simulink model "NEW_MAIN"  (R2017b)
settings: Solver=VariableStepAuto  StartTime=0.0  StopTime=10.0  RelTol=1e-3
values from neighbouring files (symbols this model uses):
  A = eye(16,16)    [full_input_list.m]
  B = zeros(16,1)    [full_input_list.m]
  C = blkdiag(eye(3,3),zeros(3,3),eye(10,10))    [full_input_list.m]
  currentMax_B = [0;0.8;0.2]    [full_input_list.m]
  deltaT = 0.00001    (= 1e-05)    [full_input_list.m]
  epsilon_UD_slew = .01    (= 0.01)    [full_input_list.m]
  epsilon_UD_spinUp = .01    (= 0.01)    [full_input_list.m]
  freq = 80    [full_input_list.m]    (also in initSimulink.m)
  H = C    [full_input_list.m]
  I_UD = [0.032808359, 0.000617048, 0.000049185;      0.000617048, 0.032531573, 0.000060042;      0.000049185, 0.000060042, 0.007799591]    [full_input_list.m]
  kd = 0.5    [full_input_list.m]    (also in initACS.m = 0.01)
  kd_UD_detumble = 6e-3    (= 0.006)    [full_input_list.m]
  kp = 1    [full_input_list.m]    (also in initACS.m = 0.01)
  magMomentMax_B = sat2CoilArea.*sat2n.*currentMax_B    [full_input_list.m]
  omega_cmd_N = 1e-1*[1 1 -.6]'    [full_input_list.m]
  omega_spinUp_MAG = 0.05    [full_input_list.m]
  OpModes = [0 0 0]    [full_input_list.m]
  OpTimes = [0 1 2]    [full_input_list.m]
  q4_cmd_init = [q4_cmd_init(2:4); q4_cmd_init(1)]    [full_input_list.m]
  Q_k = zeros(16,16)    [full_input_list.m]
  R = R_k    [full_input_list.m]
  sat2CoilArea = 0.8*[0.02; 0.02; 0.01]    [full_input_list.m]
  sat2n = [0; 100; 100]    [full_input_list.m]
  sat2Resistance = sat2WireLength.*sat2WireResistivity./sat2WireArea    [full_input_list.m]
  SeperationTime = 30000    [full_input_list.m]
  spinAxis_B = [1 0 0]    [full_input_list.m]
  u_k = zeros(16,1)    [full_input_list.m]
  w_k = zeros(16,1)    [full_input_list.m]
  Z_k = zeros(16,1)    [full_input_list.m]
undefined symbols (not defined in the file or in its folder): B_n, B_N, DiscIntNeverNeededParam, G_igrf, gyro_DCM_BS, H_igrf, I_B, IAU, Kschmidt, mag_variance, Orbit_time, R_mean, r_n, r_N, v_n, v_N
libraries: aerolibutil x48, vrlib x37, simulink x22, SimMainLibrary x20, dspmathops x6, sharedtransform x4, dspinverses x2, dspmtrx3 x1, aerolibtransform2 x1, aerolibgravity2 x1, lib_violet_env x1
(part 2 of 3)

== system NEW_MAIN/Flight Computers/Center Cube Controller/Torque Coil Management ==
  note: Why does torque coils suddenly become PWM?
  B_N : Inport
  torque_cmd_N : Inport  Port=2
  q : Inport  Port=3
  Calculate Coil Torque and Current : Subsystem
  Constant4 : Constant  Value=sat2CoilArea.*sat2n.*currentMax_B
  Magnetic Moment Unit Vector : Subsystem
  Magnetic Moment Vector : Subsystem
  Product2 : Product
  Quaternion Rotation : aerolibutil/Quaternion Rotation
  Reduce Wasted Effort : Subsystem
  Saturation : Saturate  Commented=on  UpperLimit=magMomentMax_B(2:3)  LowerLimit=-magMomentMax_B(2:3)
  Selector : Selector  InputPortWidth=3  IndexOptions=Index vector (dialog)  Indices=[2 3]  OutputSizes=1
  Vector Saturation1 : SimMainLibrary/Vector Saturation
      settings: SourceProductName=CUGravity Library
  torque : Constant  Commented=on  Value=[0;1;-1]
  torque_coils : Outport
  CenterCube_PWM_cmds : Outport  Port=2
  wires:
  Constant4/1 -> Selector/1
  B_N/1 -> Calculate Coil Torque and Current/4(B_N), Quaternion Rotation/2
  q/1 -> Quaternion Rotation/1, Calculate Coil Torque and Current/3(q), Magnetic Moment Unit Vector/2(q)
  Reduce Wasted Effort/1(mu_sat_B1) -> Calculate Coil Torque and Current/2(mu_B23)  "mu_B23"
  Vector Saturation1/1 -> Reduce Wasted Effort/2(mu_sat_B)  "mu_sat_B"
  torque_cmd_N/1 -> Magnetic Moment Vector/2(torque_cmd_N), Calculate Coil Torque and Current/1(torque_cmd_N), Magnetic Moment Unit Vector/1(torque_cmd_N)  "torque_cmd_N"
  Magnetic Moment Unit Vector/1(muHat_B) -> Magnetic Moment Vector/1(muHat_B), Reduce Wasted Effort/1(muHat_B)
  Quaternion Rotation/1 -> Reduce Wasted Effort/3(B_B), Magnetic Moment Vector/3(B_B)  "B_B"
  Product2/1 -> torque_coils/1
  Magnetic Moment Vector/1(mu_raw_B) -> Vector Saturation1/1  "mu_raw_B"
  Calculate Coil Torque and Current/1(torque_N) -> Product2/1
  Calculate Coil Torque and Current/2(Sign_B & mu) -> Product2/2
  Calculate Coil Torque and Current/3(coils_I) -> CenterCube_PWM_cmds/1
  Selector/1 -> Vector Saturation1/2

== system NEW_MAIN/Flight Computers/CenterCube EKF/Kalman Gain and Estamated State Computation ==
  P_kp : Inport
  x_kp : Inport  Port=2
  Y : Inport  Port=3
  " LU Inverse" : dspinverses/ LU Inverse
      settings: SourceProductName=DSP System Toolbox
  Add1 : Sum
  Add2 : Sum
  Add3 : Sum  Inputs=-+
  H : Constant  Value=H
  H1 : Constant  Value=H
  Math Function : Math  Operator=transpose  SaturateOnIntegerOverflow=on
  Product{,1,3..4,6} (5 alike) : Product  Multiplication=Matrix(*)
  Product2 : Product
  R : Constant  Value=R
  K : Outport
  x_k : Outport  Port=2
  wires:
  H/1 -> Product3/1, Product1/2, Math Function/1
  " LU Inverse"/1 -> Product/2
  Product1/1 -> Product/1
  Math Function/1 -> Product4/2
  Product/1 -> Product2/1, K/1  "Kalman Gain K"
  x_kp/1 -> Add2/1, Product6/2
  Y/1 -> Add3/2
  R/1 -> Add1/2
  Product4/1 -> Add1/1
  Add1/1 -> " LU Inverse"/1
  Product3/1 -> Product4/1
  H1/1 -> Product6/1
  Product6/1 -> Add3/1
  P_kp/1 -> Product3/2, Product1/1
  Add2/1 -> x_k/1
  Add3/1 -> Product2/2
  Product2/1 -> Add2/2

== system NEW_MAIN/Flight Computers/CenterCube EKF/New State Prediction  ==
  note: LKF
  note: EKF
  P_k-1 : Inport
  x_k-1 : Inport  Port=2
  A_LKF : Subsystem
  Add1 : Sum  Inputs=+++
  Add2 : Sum
  Add3 : Sum
  B : Constant  Value=B
  Math Function : Math  Operator=transpose  SaturateOnIntegerOverflow=on
  Math Function1 : Math  Operator=transpose  SaturateOnIntegerOverflow=on
  Predictions : MATLAB Function  TreatAsAtomicUnit=on
  Product{,1..5} (6 alike) : Product  Multiplication=Matrix(*)
  Q_k : Constant  Value=Q_k
  Q_k1 : Constant  Value=Q_k
  Terminator2 : Terminator
  Terminator3 : Terminator
  u_k : Constant  Value=u_k
  w_k : Constant  Value=w_k
  P_kp : Outport
  "x_kp  " : Outport  Port=2
  wires:
  Product2/1 -> Product3/1
  Math Function/1 -> Product3/2
  Product/1 -> Add1/1
  B/1 -> Product1/1
  Product1/1 -> Add1/2
  u_k/1 -> Product1/2
  w_k/1 -> Add1/3
  Q_k/1 -> Add2/2
  P_k-1/1 -> [A], Product2/2
  Product3/1 -> Add2/1
  x_k-1/1 -> Predictions/1(x_ko), Product/2, A_LKF/1(In1)
  A_LKF/1(Out1) -> Product2/1, Math Function/1, Product/1  "A"
  Predictions/1(F) -> Math Function1/1, Product4/1
  [A] -> Product4/2
  Product4/1 -> Product5/1
  Math Function1/1 -> Product5/2
  Predictions/2(x_kp) -> "x_kp  "/1  "x_kps"
  Product5/1 -> Add3/1
  Q_k1/1 -> Add3/2
  Add3/1 -> P_kp/1  "P_kp"
  Add2/1 -> Terminator2/1  "P_kp"
  Add1/1 -> Terminator3/1  "x_kp"

== system NEW_MAIN/Flight Computers/CenterCube EKF/Y computation ==
  In1 : Inport
  Add2 : Sum
  C : Constant  Value=C
  Product2 : Product  Multiplication=Matrix(*)
  "Z_k " : Constant  Value=Z_k
  Y : Outport
  wires:
  Add2/1 -> Y/1
  "Z_k "/1 -> Add2/2
  In1/1 -> Product2/2
  C/1 -> Product2/1
  Product2/1 -> Add2/1

== system NEW_MAIN/Flight Computers/CenterCube EKF/x_measured ==
  Sensor_data : Inport
  Bus Selector1 : BusSelector  OutputSignals=w_BN_1,magnetometer_1,sun_B,r_LLA,accelerometer_1,time
  Constant : Constant  Value=[0;0;0]
  Lookup Tables : Subsystem
  Terminator : Terminator
  Vector Concatenate : Concatenate  NumInputs=5
  q_N from Sensors : Subsystem
  x_measured : Outport
  B_N : Outport  Port=2
  wires:
  Bus Selector1/4 -> Vector Concatenate/1, Lookup Tables/1(x_pos)  "<r_LLA>"
  Vector Concatenate/1 -> x_measured/1
  Lookup Tables/2(V_sun_N) -> q_N from Sensors/4(V_sun_N)
  Bus Selector1/3 -> q_N from Sensors/2(V_sun_B)  "<sun_B>"
  Lookup Tables/1(B_N) -> B_N/1, q_N from Sensors/3(B_N)
  q_N from Sensors/2(Q) -> Terminator/1
  Sensor_data/1 -> Bus Selector1/1
  Bus Selector1/1 -> Vector Concatenate/4  "<w_BN_1>"
  Constant/1 -> Vector Concatenate/2  "xdot_measured"
  Bus Selector1/5 -> Vector Concatenate/3  "<accelerometer_1>"
  q_N from Sensors/1(q_N) -> Vector Concatenate/5  "quat_measured"
  Bus Selector1/2 -> q_N from Sensors/1(B_B)  "<magnetometer_1>"
  Bus Selector1/6 -> Lookup Tables/2(time)  "<time>"

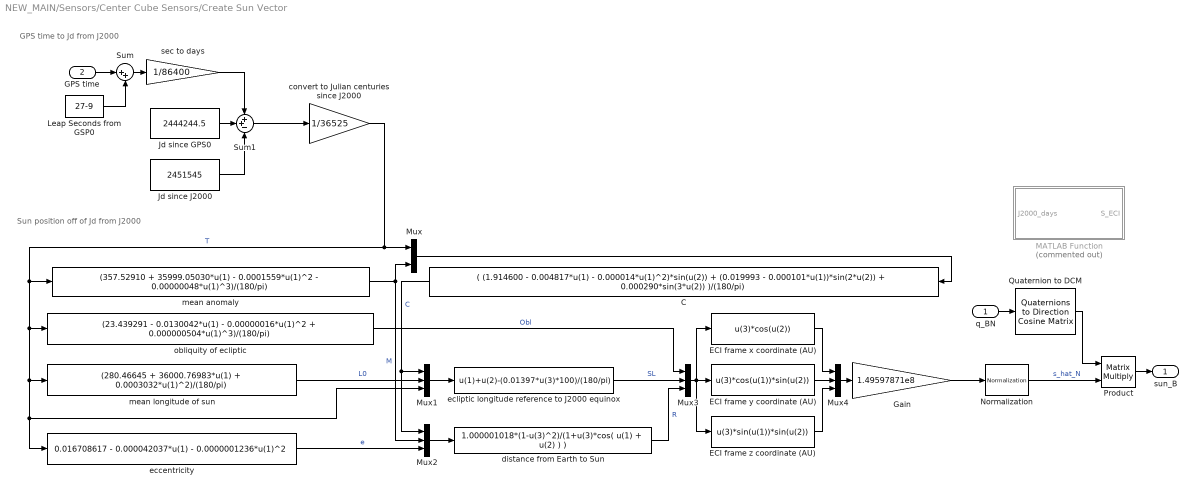
== system NEW_MAIN/Sensors/Center Cube Sensors/Create Sun Vector ==
  note: Sun position off of
      | Jd from J2000
  note: GPS time to
      | Jd from J2000
  q_BN : Inport
  GPS time : Inport  Port=2
  C : Fcn  Expr=( (1.914600 - 0.004817*u(1) - 0.000014*u(1)^2)*sin(u(2)) + (0.019993 - 0.000101*u(1))*sin(2*u(2)) + 0.000290*sin(3*u(2)) )/(180/pi)
  "ECI frame x coordinate (AU) " : Fcn  Expr=u(3)*cos(u(2))
  "ECI frame y coordinate (AU) " : Fcn  Expr=u(3)*cos(u(1))*sin(u(2))
  "ECI frame z coordinate (AU) " : Fcn  Expr=u(3)*sin(u(1))*sin(u(2))
  Gain : Gain  Gain=1.49597871e8
  Jd since GPS0 : Constant  Value=2444244.5
  Jd since J2000 : Constant  Value=2451545
  "Leap Seconds from GSP0 " : Constant  Value=27-9
  MATLAB Function : MATLAB Function  Commented=on  TreatAsAtomicUnit=on
  Mux : Mux  Inputs=2
  Mux{1..4} (4 alike) : Mux  Inputs=3
  Normalization : dspmathops/Normalization  NormType=2-norm  Bias=1e-10  NormOver=Each column  Dimension=1  outputDataTypeStr=Inherit: Same as product output  outputLastDataTypeStr=Inherit: Same as product output  outputMin=[]  outputMax=[]  accumDataTypeStr=Inherit: Same as product output  accumLastDataTypeStr=Inherit: Same as product output  roundingMode=Floor  overflowMode=off
      settings: SourceProductName=DSP System Toolbox
  Product : Product  Multiplication=Matrix(*)
  Quaternion to DCM : sharedtransform/Quaternions to  Direction Cosine Matrix
      settings: SourceProductName=Aerospace Blockset  SourceProductBaseCode=AE
  Sum : Sum  Inputs=|++
  Sum1 : Sum  Inputs=++-
  convert to Julian centuries since J2000 : Gain  Gain=1/36525
  distance from Earth to Sun : Fcn  Expr=1.000001018*(1-u(3)^2)/(1+u(3)*cos( u(1) + u(2) ) )
  eccentricity : Fcn  Expr=0.016708617 - 0.000042037*u(1) - 0.0000001236*u(1)^2
  ecliptic longitude reference to J2000 equinox : Fcn  Expr=u(1)+u(2)-(0.01397*u(3)*100)/(180/pi)
  mean anomaly : Fcn  Expr=(357.52910 + 35999.05030*u(1) - 0.0001559*u(1)^2 - 0.00000048*u(1)^3)/(180/pi)
  mean longitude of sun : Fcn  Expr=(280.46645 + 36000.76983*u(1) + 0.0003032*u(1)^2)/(180/pi)
  obliquity of ecliptic : Fcn  Expr=(23.439291 - 0.0130042*u(1) - 0.00000016*u(1)^2 + 0.000000504*u(1)^3)/(180/pi)
  sec to days : Gain  Gain=1/86400
  sun_B : Outport
  wires:
  Product/1 -> sun_B/1
  q_BN/1 -> Quaternion to DCM/1
  Normalization/1 -> Product/2  "s_hat_N"
  Quaternion to DCM/1 -> Product/1
  Gain/1 -> Normalization/1
  Jd since J2000/1 -> Sum1/3
  Jd since GPS0/1 -> Sum1/2
  sec to days/1 -> Sum1/1
  Sum/1 -> sec to days/1
  "Leap Seconds from GSP0 "/1 -> Sum/2
  GPS time/1 -> Sum/1
  Mux3/1 -> "ECI frame z coordinate (AU) "/1, "ECI frame y coordinate (AU) "/1, "ECI frame x coordinate (AU) "/1
  obliquity of ecliptic/1 -> Mux3/1  "Obl"
  distance from Earth to Sun/1 -> Mux3/3  "R"
  Mux2/1 -> distance from Earth to Sun/1
  ecliptic longitude reference to J2000 equinox/1 -> Mux3/2  "SL"
  eccentricity/1 -> Mux2/3  "e"
  mean anomaly/1 -> Mux2/2, Mux/2  "M"
  C/1 -> Mux2/1, Mux1/1  "C"
  Mux1/1 -> ecliptic longitude reference to J2000 equinox/1
  Mux/1 -> C/1
  mean longitude of sun/1 -> Mux1/2  "L0"
  convert to Julian centuries since J2000/1 -> eccentricity/1, Mux1/3, mean longitude of sun/1, obliquity of ecliptic/1, mean anomaly/1, Mux/1  "T"
  Sum1/1 -> convert to Julian centuries since J2000/1
  "ECI frame y coordinate (AU) "/1 -> Mux4/2
  "ECI frame x coordinate (AU) "/1 -> Mux4/1
  "ECI frame z coordinate (AU) "/1 -> Mux4/3
  Mux4/1 -> Gain/1

== system NEW_MAIN/Sensors/Center Cube Sensors/GPS ==
  note: Position in the sensor reference frame
  note: GPS Sensor Spoofing
      | We must specify the GPS variance and seed later when we have more time
      |
      | DCM of ECFE wrt ECI is not filled in
      |
      | GPS start time needs to be filled in.
      |
      | Violet was able to check for corrupt signals - that is the next step
  note: Velocity in the sensor reference frame
  r_N : Inport
  v_N : Inport  Port=2
  DCM of ECFC wrt ECI : Constant  Value=eye(3)
  DCM of ECFC wrt ECI1 : Constant  Value=eye(3)
  Digital Clock : DigitalClock
  GPS start time : Constant  Value=0
  Position random noise : RandomNumber  SampleTime=0.1
  Product : Product
  Product1 : Product
  Sum : Sum
  Sum1 : Sum
  Sum2 : Sum  Inputs=|++
  Velocity random noise : RandomNumber  SampleTime=0.1
  r_S : Outport
  v_S : Outport  Port=2
  Time : Outport  Port=3
  wires:
  Sum/1 -> r_S/1
  Position random noise/1 -> Sum/2
  Sum1/1 -> v_S/1
  Velocity random noise/1 -> Sum1/2
  GPS start time/1 -> Sum2/1
  Digital Clock/1 -> Sum2/2
  Sum2/1 -> Time/1
  DCM of ECFC wrt ECI/1 -> Product/1
  r_N/1 -> Product/2
  Product/1 -> Sum/1
  DCM of ECFC wrt ECI1/1 -> Product1/1
  v_N/1 -> Product1/2
  Product1/1 -> Sum1/1

== system NEW_MAIN/Sensors/Center Cube Sensors/Gyro ==
  note: Gyro Sensor Spoofing
      |
      | Lots of work left to be done on the Gyro. Violet tracks the gyro bias - necessary?
      |
      | Violet also records the time of the gyro - is this simply a diagnostic step?
  w_BN_B : Inport
  Bias : MATLAB Function  TreatAsAtomicUnit=on
  Bus Creator : BusCreator  Inputs=2
  Digital Clock : DigitalClock
  Discrete-Time Integrator : DiscreteIntegrator  gainval=1  InitialConditionSetting=State (most efficient)  ICPrevOutput=DiscIntNeverNeededParam  ICPrevScaledInput=DiscIntNeverNeededParam
  Gyro_DCM_BS : Constant  Value=gyro_DCM_BS
  Product : Product  Multiplication=Matrix(*)
  Random Bias Steps : RandomNumber  SampleTime=0.1
  Random Noise : RandomNumber  SampleTime=0.1
  Sum : Sum
  w_SN_S_m : Outport
  time : Outport  Port=2
  Gyro : Outport  Port=3
  wires:
  w_BN_B/1 -> Product/2
  Random Bias Steps/1 -> Discrete-Time Integrator/1
  Product/1 -> Sum/1
  Discrete-Time Integrator/1 -> Sum/2
  Sum/1 -> Bias/1(w)
  Random Noise/1 -> Bias/2(noise)
  Bias/1(wn) -> Bus Creator/1, w_SN_S_m/1
  Gyro_DCM_BS/1 -> Product/1
  Digital Clock/1 -> Bus Creator/2, time/1
  Bus Creator/1 -> Gyro/1

== system NEW_MAIN/Sensors/Center Cube Sensors/Magnetometer ==
  note: Teslas to Gauss
  note: from r_E to b_B is in Violet Dynamics Block.
      | The rest is in their sensor block.
  note: b_B
  note: DCM of Body wrt Neutral
  note: Pulled from NASA Langley
  note: The block takes the magnetic field in the body reference frame
      | and transforms it into magnetic field in the sensor reference
      | frame.
      |
      | We still need the DCM and the variance of the magnetometer
  r_E : Inport  PortDimensions=[1 3]
  Bus Creator : BusCreator  Inputs=2
  DCM B wrt S : Constant  Value=eye(3)
  DCM of BN : Constant  Value=eye(3)
  DCM of ECFC wrt ECI : Constant  Value=eye(3)
  Digital Clock : DigitalClock
  Gain : Gain  Gain=1e4
  Magnetic Field Model : Subsystem
  Math Function : Math  Operator=transpose  SaturateOnIntegerOverflow=on
  Math Function1 : Math  Operator=transpose  SaturateOnIntegerOverflow=on
  Matrix Multiply : Product  Multiplication=Matrix(*)
  Matrix Multiply1 : Product  Multiplication=Matrix(*)
  Product : Product  Multiplication=Matrix(*)
  Random Number : RandomNumber  Variance=mag_variance  SampleTime=0.1
  Sine Wave : Sin  Amplitude=0 * 1e-6 * randn(3, 1)  Frequency=2*pi / (90 * 60)  SampleTime=0
  Sum : Sum  Inputs=|++
  Sum1 : Sum  Inputs=|++
  b_S : Outport
  Time : Outport  Port=2
  Magnetometer : Outport  Port=3
  wires:
  Matrix Multiply1/1 -> Sum/1
  Random Number/1 -> Sum/2
  DCM B wrt S/1 -> Math Function/1
  Sum/1 -> Product/2
  Math Function/1 -> Product/1
  Product/1 -> Gain/1
  Gain/1 -> Bus Creator/1, b_S/1
  r_E/1 -> Magnetic Field Model/1(r_E)
  Magnetic Field Model/1(b_E) -> Sum1/1
  Sine Wave/1 -> Sum1/2
  Sum1/1 -> Matrix Multiply/2
  Math Function1/1 -> Matrix Multiply/1
  Matrix Multiply/1 -> Matrix Multiply1/2
  DCM of ECFC wrt ECI/1 -> Math Function1/1
  DCM of BN/1 -> Matrix Multiply1/1
  Digital Clock/1 -> Bus Creator/2, Time/1
  Bus Creator/1 -> Magnetometer/1

== system NEW_MAIN/Sensors/Center Cube Sensors/Sun Sensor ==
  In1 : Inport
  Out1 : Outport
  wires:
  In1/1 -> Out1/1

== system NEW_MAIN/Flight Computers/Center Cube Controller/SafeMode/STATUS_MODE_DETERMINATION/ATTITUDE_COMPENSATOR_OLD.TorqueD ==
  note: Regulator
      | - q_target = <input>
      | - w_target = [0 0 0]
  note: Derivative Controller
      | This controller is a pure derivative controller. It calculates torque to purely oppose the angular velocity. It is better behaved in the short-run than a PD controller projected onto the B field normal plane, but it does not allow for a quaternion command, only a detumble to an unknown attitude.
  note: Markley Regulator
      | This regulator takes the current directional quaterion vector, the target quaterion, the intertial matrix, and the current angular velocity to determine the required torque necessary to the slew.
      |
      | The equation is 7.8 listed on page 290 of Fundamentals of Spacecraft Attitude Determination and Control. The input I is currently not defined. Also important to the equation is equation 7.2
  w_BN_N : Inport
  I_B : Inport  Port=2
  q : Inport  Port=3
  f : TriggerPort  TriggerType=function-call  VariantControl=(inherit)
      settings: CopyFcn=Stateflow.SLINSF.SimulinkMan.removeBlockPreDeleteFcn  PreDeleteFcn=Stateflow.SLINSF.SimulinkMan.unsafePredeleteFcn
  Display : Display
  Display3 : Display
  Gain3 : Gain  Gain=kd_UD_detumble
  Gain5 : Gain  Gain=-1
  Gain6 : Gain  Commented=on  Gain=1/I_B(1,1)
  Math Function : Math  Operator=transpose  SaturateOnIntegerOverflow=on
  Product2 : Product  Multiplication=Matrix(*)
  Product3 : Product  Inputs=3  Multiplication=Matrix(*)
  Q_B_N : Display
  Quaternions to Direction Cosine Matrix : sharedtransform/Quaternions to  Direction Cosine Matrix
      settings: SourceProductName=Aerospace Blockset  SourceProductBaseCode=AE
  Scope : Scope
  T_N : Outport
  wires:
  Math Function/1 -> Product3/1
  q/1 -> Quaternions to Direction Cosine Matrix/1, Scope/1
  Product3/1 -> Product2/1, Display/1  "I_N"
  Quaternions to Direction Cosine Matrix/1 -> Q_B_N/1, Product3/3, Math Function/1
  Gain3/1 -> T_N/1  "torque_N"
  I_B/1 -> Product3/2, Display3/1
  Gain5/1 -> Gain3/1
  w_BN_N/1 -> Product2/2  "w_BN_N"
  Product2/1 -> Gain5/1

== system NEW_MAIN/Flight Computers/Center Cube Controller/SafeMode/STATUS_MODE_DETERMINATION/ATTITUDE_COMPENSATOR_OLD.TorqueDeployed ==
  note: Regulator
      | - q_target = [0 0 0 1]
      | - w_target = [0 0 0]
  q : Inport
  w_BN_N : Inport  Port=2
  f : TriggerPort  TriggerType=function-call  VariantControl=(inherit)
      settings: CopyFcn=Stateflow.SLINSF.SimulinkMan.removeBlockPreDeleteFcn  PreDeleteFcn=Stateflow.SLINSF.SimulinkMan.unsafePredeleteFcn
  Add : Sum
  Gain : Gain  Gain=-1
  Gain1 : Gain  Gain=kp
  Gain2 : Gain  Gain=-1
  Gain3 : Gain  Gain=kd
  Quaternion Inverse : aerolibutil/Quaternion Inverse
      settings: SourceProductName=Aerospace Blockset
  Quaternion Multiplication : aerolibutil/Quaternion Multiplication
  Selector : Selector  InputPortWidth=4  IndexOptions=Index vector (dialog)  Indices=[1 2 3]  OutputSizes=1
  Target q : Constant  Value=[ 0 0 0 1 ]
  T_N : Outport
  wires:
  Gain1/1 -> Gain/1
  Gain2/1 -> Add/2
  Gain/1 -> Add/1
  w_BN_N/1 -> Gain3/1
  Quaternion Inverse/1 -> Quaternion Multiplication/2
  Gain3/1 -> Gain2/1
  Add/1 -> T_N/1
  q/1 -> Quaternion Multiplication/1
  Selector/1 -> Gain1/1
  Quaternion Multiplication/1 -> Selector/1
  Target q/1 -> Quaternion Inverse/1

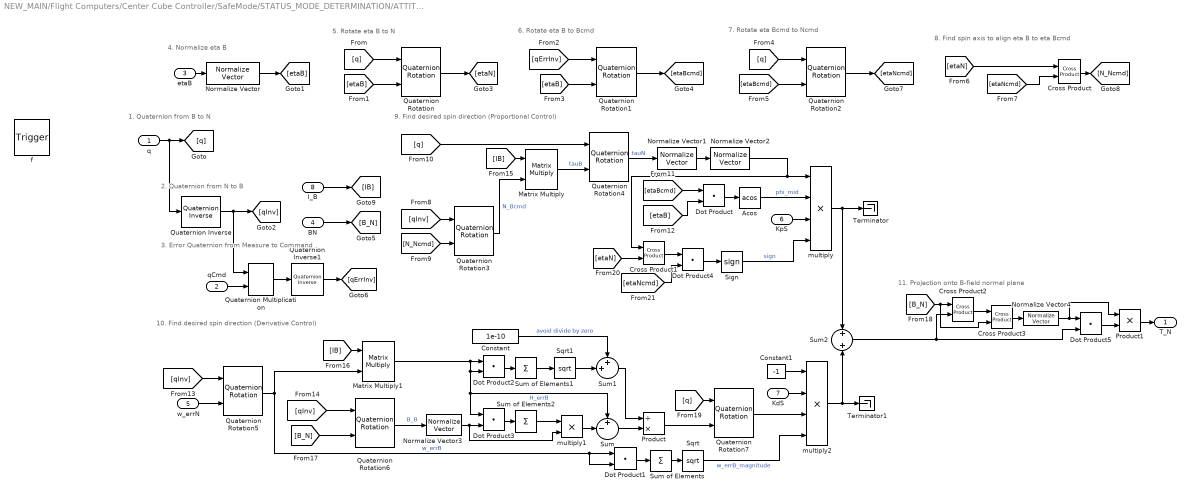
== system NEW_MAIN/Flight Computers/Center Cube Controller/SafeMode/STATUS_MODE_DETERMINATION/ATTITUDE_COMPENSATOR_OLD.TorquePD_Slew ==
  note: 9. Find desired spin direction (Proportional Control)
  note: 10. Find desired spin direction (Derivative Control)
  note: 4. Normalize eta B
  note: 5. Rotate eta B to N
  note: 6. Rotate eta B to Bcmd
  note: 7. Rotate eta Bcmd to Ncmd
  note: 8. Find spin axis to align eta B to eta Bcmd
  note: 1. Quaternion from B to N
  note: 3. Error Quaternion from Measure to Command
  note: 2. Quaternion from N to B
  note: 11. Projection onto B-field normal plane
  q : Inport
  qCmd : Inport  Port=2
  etaB : Inport  Port=3
  BN : Inport  Port=4
  w_errN : Inport  Port=5
  KpS : Inport  Port=6
  KdS : Inport  Port=7
  I_B : Inport  Port=8
  f : TriggerPort  TriggerType=function-call  VariantControl=(inherit)
      settings: CopyFcn=Stateflow.SLINSF.SimulinkMan.removeBlockPreDeleteFcn  PreDeleteFcn=Stateflow.SLINSF.SimulinkMan.unsafePredeleteFcn
  Acos : Trigonometry  Operator=acos
  Constant : Constant  Value=1e-10
  Constant1 : Constant  Value=-1
  Cross Product{,1..3} (4 alike) : vrlib/Utilities/Cross Product
      settings: SourceProductBaseCode=VR
  Dot Product{,1..5} (6 alike) : DotProduct  InputSameDT=on  OutDataTypeStr=Inherit: Inherit via internal rule
  Matrix Multiply : Product  Multiplication=Matrix(*)
  Matrix Multiply1 : Product  Multiplication=Matrix(*)
  Normalize Vector{,1..4} (5 alike) : vrlib/Utilities/Normalize Vector  maxzero=0
      settings: SourceProductName=Simulink 3D Animation  SourceProductBaseCode=VR
  Product : Product  Inputs=/*
  Product1 : Product
  Quaternion Inverse : aerolibutil/Quaternion Inverse
      settings: SourceProductName=Aerospace Blockset
  Quaternion Inverse1 : aerolibutil/Quaternion Inverse
      settings: SourceProductName=Aerospace Blockset
  Quaternion Multiplication : aerolibutil/Quaternion Multiplication
  Quaternion Rotation{,1..7} (8 alike) : aerolibutil/Quaternion Rotation
  Sign : Signum
  Sqrt : Sqrt  SaturateOnIntegerOverflow=on
  Sqrt1 : Sqrt  SaturateOnIntegerOverflow=on
  Sum : Sum  Inputs=+-|
  Sum of Elements : Sum  Inputs=+
  Sum of Elements1 : Sum  Inputs=+
  Sum of Elements2 : Sum  Inputs=+
  Sum1 : Sum  Inputs=++|
  Sum2 : Sum
  Terminator : Terminator
  Terminator1 : Terminator
  multiply : Product  Inputs=****
  multiply1 : Product  Inputs=**
  multiply2 : Product  Inputs=****
  T_N : Outport
  wires:
  Cross Product2/1 -> Cross Product3/1
  etaB/1 -> Normalize Vector/1
  Sqrt/1 -> multiply2/4  "w_errB_magnitude"
  [etaBcmd] -> Dot Product/1
  Sum1/1 -> Product/1
  Normalize Vector4/1 -> Product1/1, Dot Product5/1
  multiply/1 -> Terminator/1, Sum2/1
  Sum/1 -> Product/2
  Quaternion Rotation5/1 -> Dot Product1/1, Dot Product1/2, Matrix Multiply1/2  "w_errB"
  multiply2/1 -> Terminator1/1, Sum2/2
  Sign/1 -> multiply/4  "sign"
  Quaternion Rotation2/1 -> [etaNcmd]
  [etaNcmd] -> Dot Product4/2
  Constant1/1 -> multiply2/1
  Quaternion Rotation6/1 -> Normalize Vector3/1  "B_B"
  Sqrt1/1 -> Sum1/2
  Sum of Elements2/1 -> multiply1/1
  Sum of Elements1/1 -> Sqrt1/1
  Dot Product3/1 -> Sum of Elements2/1
  KdS/1 -> multiply2/2
  Quaternion Rotation7/1 -> multiply2/3
  Dot Product1/1 -> Sum of Elements/1
  multiply1/1 -> Sum/2
  Quaternion Rotation1/1 -> [etaBcmd]
  [q] -> Quaternion Rotation4/1
  [etaN] -> Cross Product1/2
  Constant/1 -> Sum1/1  "avoid divide by zero"
  KpS/1 -> multiply/3
  Matrix Multiply1/1 -> Sum/1, Dot Product3/1, Dot Product2/2, Dot Product2/1  "H_errB"
  Cross Product1/1 -> Dot Product4/1
  Normalize Vector1/1 -> Normalize Vector2/1
  Dot Product4/1 -> Sign/1
  Dot Product2/1 -> Sum of Elements1/1
  Dot Product/1 -> Acos/1
  Normalize Vector3/1 -> Dot Product3/2, multiply1/2
  I_B/1 -> [IB]
  [qInv] -> Quaternion Rotation5/1
  [etaB] -> Dot Product/2
  [q] -> Quaternion Rotation/1
  [IB] -> Matrix Multiply1/1
  Quaternion Rotation3/1 -> Matrix Multiply/2  "N_Bcmd"
  [q] -> Quaternion Rotation2/1
  [etaBcmd] -> Quaternion Rotation2/2
  Quaternion Multiplication/1 -> Quaternion Inverse1/1
  Normalize Vector2/1 -> Cross Product1/1, multiply/1
  [qInv] -> Quaternion Rotation6/1
  qCmd/1 -> Quaternion Multiplication/2
  q/1 -> [q], Quaternion Inverse/1
  [etaB] -> Quaternion Rotation1/2
  [etaB] -> Quaternion Rotation/2
  [N_Ncmd] -> Quaternion Rotation3/2
  Quaternion Rotation4/1 -> Normalize Vector1/1  "tauN"
  Quaternion Inverse/1 -> Quaternion Multiplication/1, [qInv]
  [qErrInv] -> Quaternion Rotation1/1
  Matrix Multiply/1 -> Quaternion Rotation4/2  "tauB"
  Cross Product/1 -> [N_Ncmd]
  [B_N] -> Quaternion Rotation6/2
  w_errN/1 -> Quaternion Rotation5/2
  [qInv] -> Quaternion Rotation3/1
  Normalize Vector/1 -> [etaB]
  Product1/1 -> T_N/1
  Quaternion Rotation/1 -> [etaN]
  Quaternion Inverse1/1 -> [qErrInv]
  BN/1 -> [B_N]
  Product/1 -> Quaternion Rotation7/2
  [etaN] -> Cross Product/1
  Acos/1 -> multiply/2  "phi_mid"
  [etaNcmd] -> Cross Product/2
  Cross Product3/1 -> Normalize Vector4/1
  [B_N] -> Cross Product2/1, Cross Product3/2
  Dot Product5/1 -> Product1/2
  [q] -> Quaternion Rotation7/1
  Sum of Elements/1 -> Sqrt/1
  [IB] -> Matrix Multiply/1
  Sum2/1 -> Cross Product2/2, Dot Product5/2

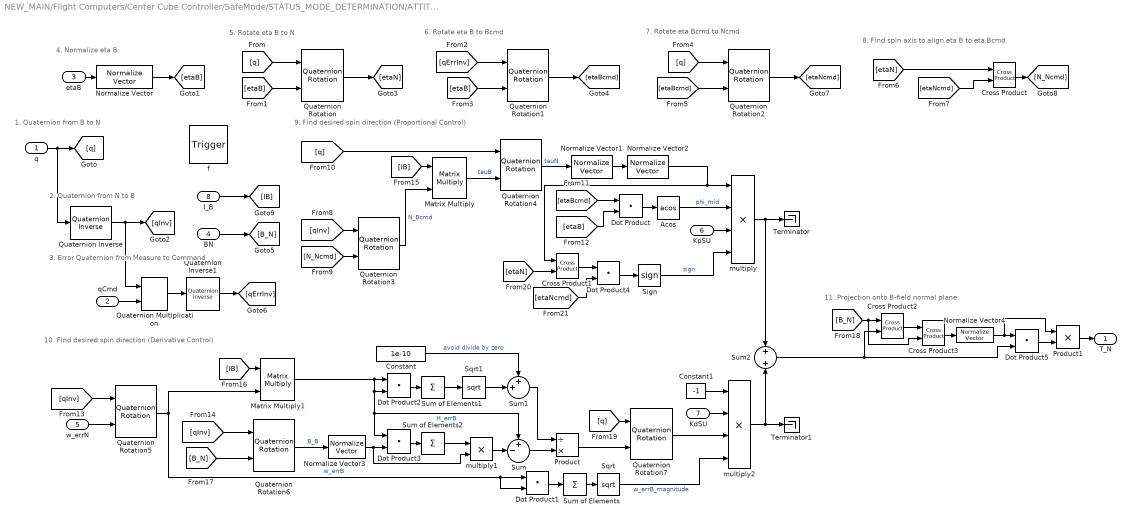
== system NEW_MAIN/Flight Computers/Center Cube Controller/SafeMode/STATUS_MODE_DETERMINATION/ATTITUDE_COMPENSATOR_OLD.TorquePD_SpinUp ==
  note: 8. Find spin axis to align eta B to eta Bcmd
  note: 9. Find desired spin direction (Proportional Control)
  note: 10. Find desired spin direction (Derivative Control)
  note: 3. Error Quaternion from Measure to Command
  note: 4. Normalize eta B
  note: 2. Quaternion from N to B
  note: 1. Quaternion from B to N
  note: 6. Rotate eta B to Bcmd
  note: 7. Rotate eta Bcmd to Ncmd
  note: 5. Rotate eta B to N
  note: 11. Projection onto B-field normal plane
  q : Inport
  qCmd : Inport  Port=2
  etaB : Inport  Port=3
  BN : Inport  Port=4
  w_errN : Inport  Port=5
  KpSU : Inport  Port=6
  KdSU : Inport  Port=7
  I_B : Inport  Port=8
  f : TriggerPort  TriggerType=function-call  VariantControl=(inherit)
      settings: CopyFcn=Stateflow.SLINSF.SimulinkMan.removeBlockPreDeleteFcn  PreDeleteFcn=Stateflow.SLINSF.SimulinkMan.unsafePredeleteFcn
  Acos : Trigonometry  Operator=acos
  Constant : Constant  Value=1e-10
  Constant1 : Constant  Value=-1
  Cross Product{,1..3} (4 alike) : vrlib/Utilities/Cross Product
      settings: SourceProductBaseCode=VR
  Dot Product{,1..5} (6 alike) : DotProduct  InputSameDT=on  OutDataTypeStr=Inherit: Inherit via internal rule
  Matrix Multiply : Product  Multiplication=Matrix(*)
  Matrix Multiply1 : Product  Multiplication=Matrix(*)
  Normalize Vector{,1..4} (5 alike) : vrlib/Utilities/Normalize Vector  maxzero=0
      settings: SourceProductName=Simulink 3D Animation  SourceProductBaseCode=VR
  Product : Product  Inputs=/*
  Product1 : Product
  Quaternion Inverse : aerolibutil/Quaternion Inverse
      settings: SourceProductName=Aerospace Blockset
  Quaternion Inverse1 : aerolibutil/Quaternion Inverse
      settings: SourceProductName=Aerospace Blockset
  Quaternion Multiplication : aerolibutil/Quaternion Multiplication
  Quaternion Rotation{,1..7} (8 alike) : aerolibutil/Quaternion Rotation
  Sign : Signum
  Sqrt : Sqrt  SaturateOnIntegerOverflow=on
  Sqrt1 : Sqrt  SaturateOnIntegerOverflow=on
  Sum : Sum  Inputs=+-|
  Sum of Elements : Sum  Inputs=+
  Sum of Elements1 : Sum  Inputs=+
  Sum of Elements2 : Sum  Inputs=+
  Sum1 : Sum  Inputs=++|
  Sum2 : Sum
  Terminator : Terminator
  Terminator1 : Terminator
  multiply : Product  Inputs=****
  multiply1 : Product  Inputs=**
  multiply2 : Product  Inputs=****
  T_N : Outport
  wires:
  Quaternion Rotation4/1 -> Normalize Vector1/1  "tauN"
  Normalize Vector2/1 -> Cross Product1/1, multiply/1
  Matrix Multiply/1 -> Quaternion Rotation4/2  "tauB"
  multiply/1 -> Terminator/1, Sum2/1
  [qInv] -> Quaternion Rotation3/1
  [etaB] -> Quaternion Rotation/2
  Quaternion Rotation5/1 -> Dot Product1/1, Dot Product1/2, Matrix Multiply1/2  "w_errB"
  [etaN] -> Cross Product/1
  KpSU/1 -> multiply/3
  Quaternion Rotation3/1 -> Matrix Multiply/2  "N_Bcmd"
  [qErrInv] -> Quaternion Rotation1/1
  [q] -> Quaternion Rotation/1
  qCmd/1 -> Quaternion Multiplication/2
  Quaternion Rotation/1 -> [etaN]
  Quaternion Rotation1/1 -> [etaBcmd]
  etaB/1 -> Normalize Vector/1
  [B_N] -> Quaternion Rotation6/2
  [B_N] -> Cross Product2/1, Cross Product3/2
  Normalize Vector3/1 -> Dot Product3/2, multiply1/2
  [etaNcmd] -> Cross Product/2
  [IB] -> Matrix Multiply/1
  Cross Product3/1 -> Normalize Vector4/1
  Product1/1 -> T_N/1
  Sum/1 -> Product/2
  Normalize Vector4/1 -> Product1/1, Dot Product5/1
  [N_Ncmd] -> Quaternion Rotation3/2
  Dot Product5/1 -> Product1/2
  Sum2/1 -> Cross Product2/2, Dot Product5/2
  Cross Product2/1 -> Cross Product3/1
  Dot Product3/1 -> Sum of Elements2/1
  [q] -> Quaternion Rotation4/1
  Sqrt/1 -> multiply2/4  "w_errB_magnitude"
  Acos/1 -> multiply/2  "phi_mid"
  Constant1/1 -> multiply2/1
  Matrix Multiply1/1 -> Sum/1, Dot Product3/1, Dot Product2/2, Dot Product2/1  "H_errB"
  Cross Product/1 -> [N_Ncmd]
  multiply2/1 -> Terminator1/1, Sum2/2
  Quaternion Rotation7/1 -> multiply2/3
  Quaternion Rotation2/1 -> [etaNcmd]
  [q] -> Quaternion Rotation2/1
  Dot Product/1 -> Acos/1
  [etaN] -> Cross Product1/2
  Normalize Vector/1 -> [etaB]
  q/1 -> [q], Quaternion Inverse/1
  w_errN/1 -> Quaternion Rotation5/2
  multiply1/1 -> Sum/2
  Sum of Elements1/1 -> Sqrt1/1
  Quaternion Inverse/1 -> Quaternion Multiplication/1, [qInv]
  [etaNcmd] -> Dot Product4/2
  [etaB] -> Dot Product/2
  Sign/1 -> multiply/4  "sign"
  Cross Product1/1 -> Dot Product4/1
  Dot Product4/1 -> Sign/1
  KdSU/1 -> multiply2/2
  [q] -> Quaternion Rotation7/1
  [qInv] -> Quaternion Rotation6/1
  Quaternion Rotation6/1 -> Normalize Vector3/1  "B_B"
  I_B/1 -> [IB]
  Sum of Elements2/1 -> multiply1/1
  Constant/1 -> Sum1/1  "avoid divide by zero"
  Dot Product2/1 -> Sum of Elements1/1
  [IB] -> Matrix Multiply1/1
  [etaBcmd] -> Dot Product/1
  [qInv] -> Quaternion Rotation5/1
  Sum of Elements/1 -> Sqrt/1
  Normalize Vector1/1 -> Normalize Vector2/1
  Product/1 -> Quaternion Rotation7/2
  [etaB] -> Quaternion Rotation1/2
  Sqrt1/1 -> Sum1/2
  Quaternion Multiplication/1 -> Quaternion Inverse1/1
  Quaternion Inverse1/1 -> [qErrInv]
  Dot Product1/1 -> Sum of Elements/1
  Sum1/1 -> Product/1
  BN/1 -> [B_N]
  [etaBcmd] -> Quaternion Rotation2/2

== system NEW_MAIN/Flight Computers/Center Cube Controller/SafeMode/TORQUE_MANAGEMENT ==
  MODE : Inport
  Kp : Inport  Port=2
  Kd : Inport  Port=3
  EstState : Inport  Port=4
  B_N : Inport  Port=5
  Bus Creator : BusCreator  Inputs=2
  Bus Creator1 : BusCreator  Inputs='r_N_est','v_N_est','q_BN_est','w_BN_est'
  Bus Selector1 : BusSelector  OutputSignals=r_N_est,v_N_est,q_BN_est,w_BN_est
  Bus Selector4 : BusSelector  OutputSignals=Cube1_estState,Cube2_estState,Cube3_estState
  DEFAULT : Subsystem
  DEPLOYED : Subsystem
  DETUMBLE : Subsystem
  Determine CMD & Error : Subsystem
  Inertia : Constant  Value=I_UD
  Merge : Merge  Inputs=4
  SPIN_UP_SLEW : Subsystem
  Switch Case : SwitchCase  CaseConditions={1,2,3}
  Terminator{,1..3,12} (5 alike) : Terminator
  eta_B1 : Constant  Value=spinAxis_B
  T_N : Outport
  Safed Att. State : Outport  Port=2
  wires:
  DEPLOYED/1(T_N) -> Merge/2
  eta_B1/1 -> SPIN_UP_SLEW/5(etaB)
  Kp/1 -> SPIN_UP_SLEW/1(Kp)
  Switch Case/4 -> DEFAULT/Action
  Switch Case/3 -> DETUMBLE/Action
  Switch Case/2 -> DEPLOYED/Action
  Kd/1 -> SPIN_UP_SLEW/2(Kd)
  DETUMBLE/1(T_N) -> Merge/3
  SPIN_UP_SLEW/1(T_N) -> Merge/1
  Switch Case/1 -> SPIN_UP_SLEW/Action
  Inertia/1 -> DETUMBLE/3(I_B), SPIN_UP_SLEW/8(I_B)
  MODE/1 -> Switch Case/1
  DEFAULT/1(T_N) -> Merge/4
  Merge/1 -> T_N/1
  Determine CMD & Error/2(w_errN) -> SPIN_UP_SLEW/4(w_errN)
  Bus Selector1/1 -> Bus Creator1/1, Terminator/1  "<r_N_est>"
  Bus Selector1/4 -> Bus Creator1/4, Bus Creator/2, DETUMBLE/2(w_BN_N), DEPLOYED/2(w_BN_N), Determine CMD & Error/2(w_BN_N)  "<w_BN_est>"
  EstState/1 -> Bus Selector4/1
  Bus Selector1/2 -> Bus Creator1/2, Terminator12/1  "<v_N_est>"
  Bus Selector4/3 -> Terminator2/1  "<Cube3_estState>"
  Bus Selector4/2 -> Bus Selector1/1  "<Cube2_estState>"
  Bus Selector4/1 -> Terminator1/1  "<Cube1_estState>"
  Bus Creator/1 -> Safed Att. State/1
  Bus Creator1/1 -> Terminator3/1  "EKFAE"
  Bus Selector1/3 -> Bus Creator/1, DETUMBLE/1(q), DEPLOYED/1(q), SPIN_UP_SLEW/7(q), Determine CMD & Error/1(q), Bus Creator1/3  "<q_BN_est>"
  B_N/1 -> SPIN_UP_SLEW/6(BN)
  Determine CMD & Error/1(qCmd) -> SPIN_UP_SLEW/3(qCmd)

== system NEW_MAIN/Flight Computers/Center Cube Controller/Torque Coil Management/Calculate Coil Torque and Current ==
  torque_cmd_N : Inport
  mu_B23 : Inport  Port=2
  q : Inport  Port=3
  B_N : Inport  Port=4
  Constant : Constant  Value=0
  Cross Product1 : vrlib/Utilities/Cross Product
      settings: SourceProductBaseCode=VR
  Demux : Demux  Outputs=2
  Demux1 : Demux  Outputs=2
  Gain4 : Gain  Gain=1/sat2CoilArea(2)
  Gain5 : Gain  Gain=1/sat2n(2)
  Gain6 : Gain  Gain=1/sat2CoilArea(3)
  Gain7 : Gain  Gain=1/sat2n(3)
  Math Function : Math  Operator=transpose  SaturateOnIntegerOverflow=on
  Mux : Mux  Inputs=3
  Mux1 : Mux  Inputs=2
  Product1 : Product  Multiplication=Matrix(*)
  Product3 : Product
  Quaternion Rotation1 : aerolibutil/Quaternion Rotation
  Sign : Signum
  torque_N : Outport
  Sign_B & mu : Outport  Port=2
  coils_I : Outport  Port=3
  wires:
  mu_B23/1 -> Demux/1, Product3/2
  Constant/1 -> Mux/1
  Mux/1 -> Quaternion Rotation1/2  "mu_B"
  Demux/1 -> Mux/2
  Demux/2 -> Mux/3
  Quaternion Rotation1/1 -> Cross Product1/1  "mu_N"
  q/1 -> Quaternion Rotation1/1
  Cross Product1/1 -> torque_N/1, Product1/2  "torque_N"
  B_N/1 -> Cross Product1/2
  Product1/1 -> Sign/1
  Sign/1 -> Sign_B & mu/1, Product3/1
  Math Function/1 -> Product1/1
  torque_cmd_N/1 -> Math Function/1
  Mux1/1 -> coils_I/1
  Demux1/1 -> Gain4/1
  Product3/1 -> Demux1/1
  Gain6/1 -> Gain7/1
  Gain7/1 -> Mux1/2
  Gain5/1 -> Mux1/1
  Gain4/1 -> Gain5/1
  Demux1/2 -> Gain6/1

== system NEW_MAIN/Flight Computers/Center Cube Controller/Torque Coil Management/Magnetic Moment Unit Vector ==
  note: Aperp_B is the normal vector to the plane of attainable magnetic moments by the 2 coils in the b2 and b3 directions
  torque_cmd_N : Inport
  q : Inport  Port=2
  Aperp_B : Constant  Value=[1;0;0]
  Cross Product : vrlib/Utilities/Cross Product
      settings: SourceProductBaseCode=VR
  Display : Display  Commented=on
  Normalize Vector : vrlib/Utilities/Normalize Vector  maxzero=0
      settings: SourceProductName=Simulink 3D Animation  SourceProductBaseCode=VR
  Quaternion Rotation : aerolibutil/Quaternion Rotation
  muHat_B : Outport
  wires:
  Quaternion Rotation/1 -> Display/1, Cross Product/2  "torque_B"
  torque_cmd_N/1 -> Quaternion Rotation/2
  Normalize Vector/1 -> muHat_B/1  "muHat_B"
  Aperp_B/1 -> Cross Product/1
  q/1 -> Quaternion Rotation/1
  Cross Product/1 -> Normalize Vector/1

== system NEW_MAIN/Flight Computers/Center Cube Controller/Torque Coil Management/Magnetic Moment Vector ==
  note: Singularity aviodance algorithm is flawed. Need to redo.
  muHat_B : Inport
  torque_cmd_N : Inport  Port=2
  B_B : Inport  Port=3
  Acos : Trigonometry  Operator=acos
  Add : Sum  Inputs=++|
  Avoid singularity : Constant  Value=0
  Divide : Product  Inputs=*//
  Dot Product : DotProduct  InputSameDT=on  OutDataTypeStr=Inherit: Inherit via internal rule
  Normalize Vector1 : vrlib/Utilities/Normalize Vector  maxzero=0
      settings: SourceProductName=Simulink 3D Animation  SourceProductBaseCode=VR
  Product : Product
  Selector1 : Selector  InputPortWidth=3  IndexOptions=Index vector (dialog)  Indices=[2 3]  OutputSizes=1
  Sin : Trigonometry
  Vector Magnitude : SimMainLibrary/Vector Magnitude
      settings: SourceProductName=CUGravity Library
  Vector Magnitude1 : SimMainLibrary/Vector Magnitude
      settings: SourceProductName=CUGravity Library
  mu_raw_B : Outport
  wires:
  Vector Magnitude1/1 -> Divide/2
  Dot Product/1 -> Acos/1
  Divide/1 -> Product/1  "||mu||"
  torque_cmd_N/1 -> Vector Magnitude/1
  B_B/1 -> Normalize Vector1/1, Vector Magnitude1/1
  muHat_B/1 -> Product/2, Dot Product/2
  Sin/1 -> Add/1
  Acos/1 -> Sin/1
  Vector Magnitude/1 -> Divide/1
  Avoid singularity/1 -> Add/2
  Add/1 -> Divide/3
  Normalize Vector1/1 -> Dot Product/1
  Product/1 -> Selector1/1  "mu_rawVec_B"
  Selector1/1 -> mu_raw_B/1

== system NEW_MAIN/Flight Computers/Center Cube Controller/Torque Coil Management/Reduce Wasted Effort ==
  note: Reduce Wasted Effort
      | Author: Aaron Sandoval
      | This function detects how close the direction of the commanded mag. moment is to the external magnetic field. If it is very close, then the resulting torque will be minimal, and a lot of energy is expelled for little torque. A nonlinear, continuous gain is applied which drives the torque to zero near alignment, and preserves the value otherwise.
  muHat_B : Inport
  mu_sat_B : Inport  Port=2
  B_B : Inport  Port=3
  Constant2 : Constant  Value=100
  Dot Product : DotProduct  InputSameDT=on  OutDataTypeStr=Inherit: Inherit via internal rule
  Fcn : Fcn  Expr=1-exp(-u(2)*(u(1)+1)^2)-exp(-u(2)*(u(1)-1)^2)
  Mux2 : Mux  Inputs=2
  Normalize Vector : vrlib/Utilities/Normalize Vector  maxzero=0
      settings: SourceProductName=Simulink 3D Animation  SourceProductBaseCode=VR
  Product1 : Product
  Ramp : simulink/Sources/Ramp  Commented=on  slope=1  start=0  X0=-2
  Scope : Scope
  mu_sat_B1 : Outport
  wires:
  mu_sat_B/1 -> Product1/1
  muHat_B/1 -> Dot Product/1
  B_B/1 -> Normalize Vector/1
  Mux2/1 -> Fcn/1
  Constant2/1 -> Mux2/2
  Fcn/1 -> Scope/1, Product1/2  "mu_sat_B"
  Product1/1 -> mu_sat_B1/1  "mu_sat_B"
  Dot Product/1 -> Mux2/1
  Normalize Vector/1 -> Dot Product/2

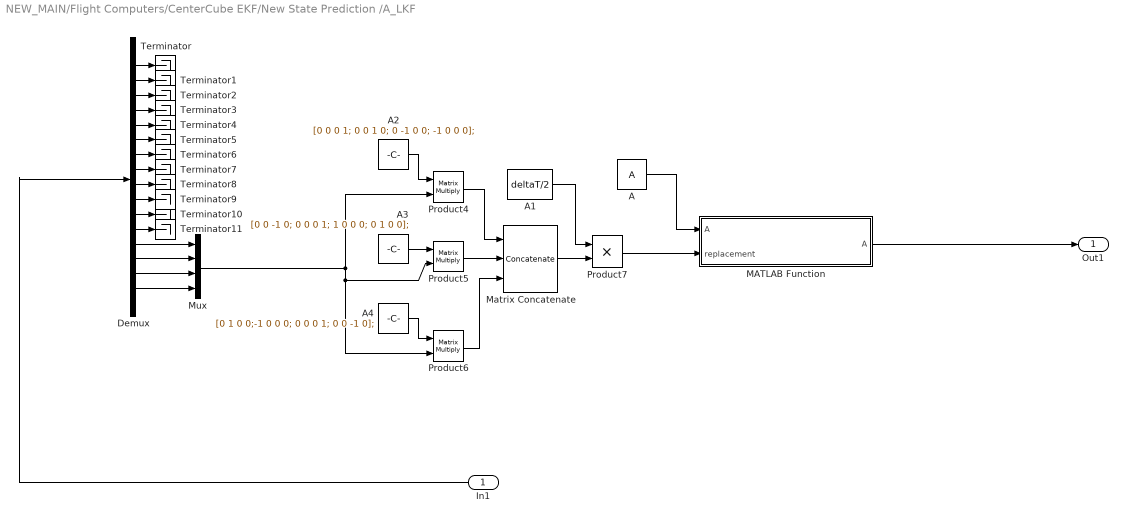
== system NEW_MAIN/Flight Computers/CenterCube EKF/New State Prediction /A_LKF ==
  In1 : Inport
  A : Constant  Value=A
  A1 : Constant  Value=deltaT/2
  A2 : Constant  Value=[0 0 0 1; 0 0 1 0; 0 -1 0 0; -1 0 0 0];
  A3 : Constant  Value=[0 0 -1 0; 0 0 0 1; 1 0 0 0; 0 1 0 0];
  A4 : Constant  Value=[0 1 0 0;-1 0 0 0; 0 0 0 1; 0 0 -1 0];
  Demux : Demux  Outputs=16
  MATLAB Function : MATLAB Function  TreatAsAtomicUnit=on
  Matrix Concatenate : Concatenate  NumInputs=3  Mode=Multidimensional array  ConcatenateDimension=2
  Mux : Mux
  Product4 : Product  Multiplication=Matrix(*)
  Product5 : Product  Multiplication=Matrix(*)
  Product6 : Product  Multiplication=Matrix(*)
  Product7 : Product
  Terminator{,1..11} (12 alike) : Terminator
  Out1 : Outport
  wires:
  In1/1 -> Demux/1
  Demux/4 -> Terminator3/1
  Demux/5 -> Terminator4/1
  Demux/3 -> Terminator2/1
  Demux/6 -> Terminator5/1
  Demux/9 -> Terminator8/1
  Demux/10 -> Terminator9/1
  Demux/7 -> Terminator6/1
  Demux/8 -> Terminator7/1
  Demux/12 -> Terminator11/1
  Demux/11 -> Terminator10/1
  Demux/13 -> Mux/1
  Demux/16 -> Mux/4
  Demux/15 -> Mux/3
  Demux/14 -> Mux/2
  Demux/1 -> Terminator/1
  Mux/1 -> Product4/2, Product6/2, Product5/2
  Product4/1 -> Matrix Concatenate/1
  A3/1 -> Product5/1
  Product6/1 -> Matrix Concatenate/3
  A4/1 -> Product6/1
  Matrix Concatenate/1 -> Product7/2
  A2/1 -> Product4/1
  Product7/1 -> MATLAB Function/2(replacement)
  MATLAB Function/1(A) -> Out1/1
  A1/1 -> Product7/1
  Product5/1 -> Matrix Concatenate/2
  Demux/2 -> Terminator1/1
  A/1 -> MATLAB Function/1("A ")

== system NEW_MAIN/Flight Computers/CenterCube EKF/x_measured/Lookup Tables ==
  note: r_N is in format:
      | - Lat (N-S) in decimal deg
      | - Long (E-W) in decimal deg
      | - Height in m
  x_pos : Inport
  time : Inport  Port=2
  Demux : Demux  Outputs=3
  ECI Position to LLA : aerolibtransform2/ECI Position to LLA  Commented=on  red=IAU-2000/2006  year=2016  month=September  day=20  hour=0  min=0  sec=0  deltaT=Sec  errorflag=Error  extraparamflag=off  eunits=Metric (MKS)  earthmodel=WGS84  flat=1/298.257223563  eqradius=6378137
      settings: AttributesFormatString=%<red>  SourceProductName=Aerospace Blockset  SourceProductBaseCode=AE
  GPS time to Jd sfrom J2000 : Subsystem
  Normalization : dspmathops/Normalization  NormType=2-norm  Bias=1e-10  NormOver=Each column  Dimension=1  outputDataTypeStr=Inherit: Same as product output  outputLastDataTypeStr=Inherit: Same as product output  outputMin=[]  outputMax=[]  accumDataTypeStr=Inherit: Same as product output  accumLastDataTypeStr=Inherit: Same as product output  roundingMode=Floor  overflowMode=off
      settings: SourceProductName=DSP System Toolbox
  "RBF!!!!! " : Constant  Value=2015
  Sun position off of Jd frm J2000 : Subsystem
  Terminator{,1..3} (4 alike) : Terminator
  World Magnetic Model 2015 : aerolibgravity2/World Magnetic Model 2015  Commented=on  units=Metric (MKS)  time_in=on  month=January  day=1  year=2015  action=Error  h_out=on  dec_out=on  inc_out=on  ti_out=on
      settings: SourceProductName=Aerospace Blockset  SourceProductBaseCode=AE
  B_N : Outport
  V_sun_N : Outport  Port=2
  wires:
  Demux/3 -> World Magnetic Model 2015/1
  Demux/1 -> World Magnetic Model 2015/2
  Demux/2 -> World Magnetic Model 2015/3
  World Magnetic Model 2015/1 -> B_N/1
  World Magnetic Model 2015/2 -> Terminator/1
  World Magnetic Model 2015/3 -> Terminator1/1
  World Magnetic Model 2015/4 -> Terminator2/1
  World Magnetic Model 2015/5 -> Terminator3/1
  x_pos/1 -> ECI Position to LLA/1
  ECI Position to LLA/1 -> Demux/1
  "RBF!!!!! "/1 -> World Magnetic Model 2015/4
  time/1 -> GPS time to Jd sfrom J2000/1(In1), ECI Position to LLA/2
  Normalization/1 -> V_sun_N/1  "s_hat_N"
  GPS time to Jd sfrom J2000/1(Out1) -> Sun position off of Jd frm J2000/1(In1)
  Sun position off of Jd frm J2000/1(Out1) -> Normalization/1

== system NEW_MAIN/Flight Computers/CenterCube EKF/x_measured/q_N from Sensors ==
  B_B : Inport
  V_sun_B : Inport  Port=2
  B_N : Inport  Port=3
  V_sun_N : Inport  Port=4
  Cross Product{1..4} (4 alike) : vrlib/Utilities/Cross Product
      settings: SourceProductBaseCode=VR
  Direction Cosine Matrix to Quaternions : sharedtransform/Direction Cosine Matrix  to Quaternions
      settings: SourceProductName=Aerospace Blockset  SourceProductBaseCode=AE
  Normalization{1..4} (4 alike) : dspmathops/Normalization  NormType=2-norm  Bias=1e-10  NormOver=Each column  Dimension=1  outputDataTypeStr=Inherit: Same as product output  outputLastDataTypeStr=Inherit: Same as product output  outputMin=[]  outputMax=[]  accumDataTypeStr=Inherit: Same as product output  accumLastDataTypeStr=Inherit: Same as product output  roundingMode=Floor  overflowMode=off
      settings: SourceProductName=DSP System Toolbox
  Product : Product  Multiplication=Matrix(*)
  Pseudoinverse : dspinverses/Pseudoinverse  wanterr=off  SimulateUsing=Interpreted execution
      settings: SourceProductName=DSP System Toolbox  SourceProductBaseCode=DS
  Vector Concatenate : Concatenate  NumInputs=3  Mode=Multidimensional array  ConcatenateDimension=2
  Vector Concatenate1 : Concatenate  NumInputs=3  Mode=Multidimensional array  ConcatenateDimension=2
  quat From DCM : MATLAB Function  Commented=on  TreatAsAtomicUnit=on
  q_N : Outport
  Q : Outport  Port=2
  wires:
  Direction Cosine Matrix to Quaternions/1 -> q_N/1
  V_sun_N/1 -> Cross Product2/1
  V_sun_B/1 -> Cross Product1/1
  B_B/1 -> Cross Product1/2, Normalization2/1
  Cross Product1/1 -> Normalization1/1
  Normalization2/1 -> Vector Concatenate1/2, Cross Product3/1  "b_2"
  Normalization1/1 -> Vector Concatenate1/3, Cross Product3/2  "b_3"
  Cross Product3/1 -> Vector Concatenate1/1  "b_1"
  B_N/1 -> Cross Product2/2, Normalization4/1
  Cross Product2/1 -> Normalization3/1
  Normalization4/1 -> Vector Concatenate/2, Cross Product4/1  "n_2"
  Normalization3/1 -> Vector Concatenate/3, Cross Product4/2  "n_3"
  Cross Product4/1 -> Vector Concatenate/1  "n_1"
  Vector Concatenate/1 -> Product/1
  Product/1 -> Direction Cosine Matrix to Quaternions/1, Q/1
  Pseudoinverse/1 -> Product/2
  Vector Concatenate1/1 -> Pseudoinverse/1

== system NEW_MAIN/Sensors/Center Cube Sensors/Magnetometer/Magnetic Field Model ==
  note: IGRF Model
      | Author: Carlos Roithmayr
  r_E : Inport  PortDimensions=[1 3]
  G : Constant  Value=G_igrf
  H : Constant  Value=H_igrf
  IGRF : lib_violet_env/IGRF Model/IGRF
  Kschmidt : Constant  Value=Kschmidt
  R_mean : Constant  Value=R_mean
  b_E : Outport  PortDimensions=3
  wires:
  IGRF/1 -> b_E/1
  R_mean/1 -> IGRF/5
  H/1 -> IGRF/3
  r_E/1 -> IGRF/1
  Kschmidt/1 -> IGRF/4
  G/1 -> IGRF/2

== system NEW_MAIN/Flight Computers/Center Cube Controller/SafeMode/TORQUE_MANAGEMENT/DEFAULT ==
  Action Port : ActionPort  ActionType=default
  Constant4 : Constant  Value=[0 0 0]
  T_N : Outport
  wires:
  Constant4/1 -> T_N/1

== system NEW_MAIN/Flight Computers/Center Cube Controller/SafeMode/TORQUE_MANAGEMENT/DEPLOYED ==
  note: Regulator
      | - q_target = [0 0 0 1]
      | - w_target = [0 0 0]
  q : Inport
  w_BN_N : Inport  Port=2
  Action Port : ActionPort  ActionType=case
  Add : Sum
  Gain1 : Gain  Gain=-1
  Gain2 : Gain  Gain=kp
  Gain3 : Gain  Gain=-1
  Gain4 : Gain  Gain=kd
  Quaternion Inverse : aerolibutil/Quaternion Inverse
      settings: SourceProductName=Aerospace Blockset
  Quaternion Multiplication : aerolibutil/Quaternion Multiplication
  Selector : Selector  InputPortWidth=4  IndexOptions=Index vector (dialog)  Indices=[1 2 3]  OutputSizes=1
  Target q : Constant  Value=[ 0 0 0 1 ]
  T_N : Outport
  wires:
  Add/1 -> T_N/1
  w_BN_N/1 -> Gain4/1
  q/1 -> Quaternion Multiplication/1
  Selector/1 -> Gain2/1
  Target q/1 -> Quaternion Inverse/1
  Quaternion Multiplication/1 -> Selector/1
  Gain3/1 -> Add/2
  Quaternion Inverse/1 -> Quaternion Multiplication/2
  Gain2/1 -> Gain1/1
  Gain1/1 -> Add/1
  Gain4/1 -> Gain3/1

== system NEW_MAIN/Flight Computers/Center Cube Controller/SafeMode/TORQUE_MANAGEMENT/DETUMBLE ==
  note: Regulator
      | - q_target = <input>
      | - w_target = [0 0 0]
  note: Derivative Controller
      | This controller is a pure derivative controller. It calculates torque to purely oppose the angular velocity. It is better behaved in the short-run than a PD controller projected onto the B field normal plane, but it does not allow for a quaternion command, only a detumble to an unknown attitude.
  note: Markley Regulator
      | This regulator takes the current directional quaterion vector, the target quaterion, the intertial matrix, and the current angular velocity to determine the required torque necessary to the slew.
      |
      | The equation is 7.8 listed on page 290 of Fundamentals of Spacecraft Attitude Determination and Control. The input I is currently not defined. Also important to the equation is equation 7.2
  q : Inport
  w_BN_N : Inport  Port=2
  I_B : Inport  Port=3
  Action Port : ActionPort  ActionType=case
  Display : Display
  Display3 : Display
  Gain3 : Gain  Gain=kd_UD_detumble
  Gain5 : Gain  Gain=-1
  Gain6 : Gain  Commented=on  Gain=1/I_B(1,1)
  Math Function : Math  Operator=transpose  SaturateOnIntegerOverflow=on
  Product2 : Product  Multiplication=Matrix(*)
  Product3 : Product  Inputs=3  Multiplication=Matrix(*)
  Q_B_N : Display
  Quaternions to Direction Cosine Matrix : sharedtransform/Quaternions to  Direction Cosine Matrix
      settings: SourceProductName=Aerospace Blockset  SourceProductBaseCode=AE
  Scope : Scope
  T_N : Outport
  wires:
  Quaternions to Direction Cosine Matrix/1 -> Q_B_N/1, Product3/3, Math Function/1
  q/1 -> Quaternions to Direction Cosine Matrix/1, Scope/1
  Gain5/1 -> Gain3/1
  w_BN_N/1 -> Product2/2
  Product2/1 -> Gain5/1
  Product3/1 -> Product2/1, Display/1  "I_N"
  Gain3/1 -> T_N/1  "torque_N"
  I_B/1 -> Product3/2, Display3/1
  Math Function/1 -> Product3/1

== system NEW_MAIN/Flight Computers/Center Cube Controller/SafeMode/TORQUE_MANAGEMENT/Determine CMD & Error ==
  q : Inport
  w_BN_N : Inport  Port=2
  Gain : Gain  Gain=omega_spinUp_MAG
  Normalize Vector : vrlib/Utilities/Normalize Vector  maxzero=0
      settings: SourceProductName=Simulink 3D Animation  SourceProductBaseCode=VR
  Quaternion Integration : Subsystem
  Quaternion Inverse : aerolibutil/Quaternion Inverse
      settings: SourceProductName=Aerospace Blockset
  Quaternion Multiplication : aerolibutil/Quaternion Multiplication
  Sum1 : Sum  Inputs=|+-
  Terminator : Terminator
  omega_N : Constant  Value=omega_cmd_N
  q_comment : Constant  Commented=on  Value=[0 0 0 1]'
  qCmd : Outport
  w_errN : Outport  Port=2
  wires:
  omega_N/1 -> Normalize Vector/1, Quaternion Integration/1(w_N)  "omega_cmd_N"
  Quaternion Integration/1(q4) -> Quaternion Inverse/1, qCmd/1
  Quaternion Inverse/1 -> Quaternion Multiplication/2
  q/1 -> Quaternion Multiplication/1
  Quaternion Multiplication/1 -> Terminator/1  "qError"
  Normalize Vector/1 -> Gain/1
  Gain/1 -> Sum1/2
  w_BN_N/1 -> Sum1/1
  Sum1/1 -> w_errN/1
